simulink model "AE_sunroof_project"  (R2022b)
settings: Solver=VariableStepAuto  StartTime=0.0  StopTime=inf  RelTol=1e-3
libraries: simulink x3
settings Model: Creator=VENKATESH  LastModifiedBy=VENKATESH

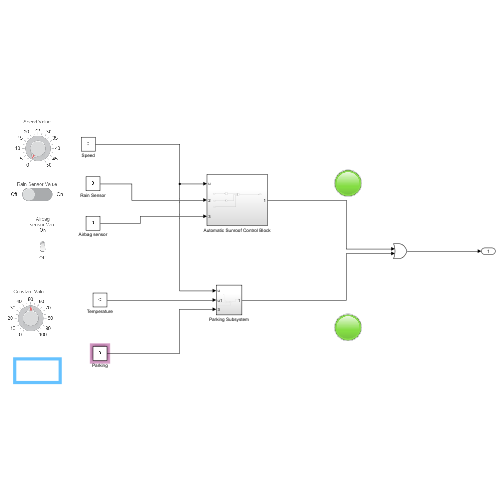
[thumbnail: Simulink's stored preview of the top-level diagram]
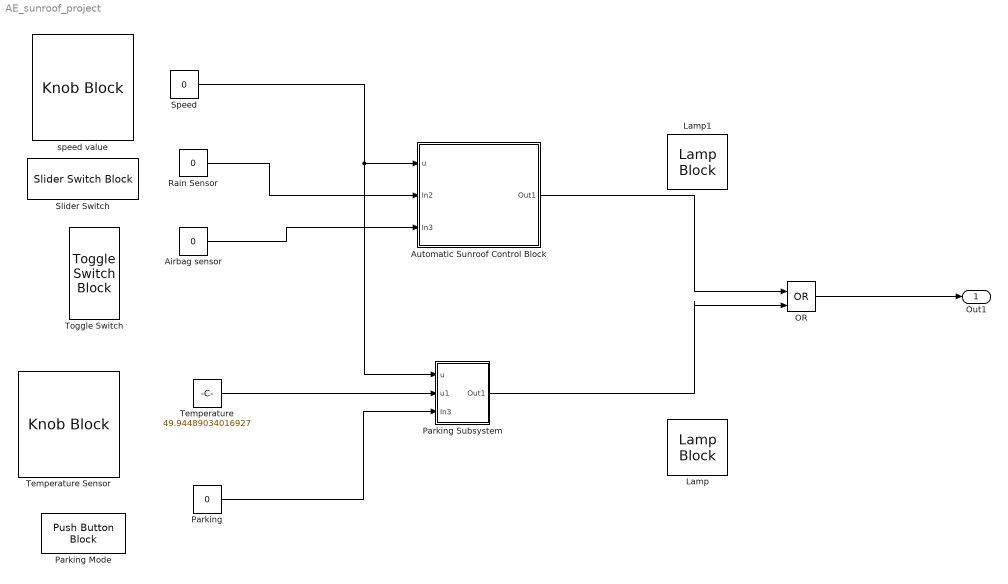
== system AE_sunroof_project ==
  Airbag sensor : Constant  Value=0
  Automatic Sunroof Control Block : Subsystem
  Lamp : LampBlock  LabelPosition=Hide
  Lamp1 : LampBlock  LabelPosition=Hide
  OR : Logic  Operator=OR  IconShape=distinctive  AllPortsSameDT=off  OutDataTypeStr=boolean
  Parking : Constant  Value=0
  Parking Mode : PushButtonBlock  ButtonType=Latch  OffValue=0.000000
  Parking Subsystem : Subsystem
  Rain Sensor : Constant  Value=0
  Slider Switch : SliderSwitchBlock
      settings: Values={{'Off', 'On'}, [0 1]}
  Speed : Constant  Value=0
  Temperature : Constant  Value=49.94489034016927
  Temperature Sensor : KnobBlock
  Toggle Switch : ToggleSwitchBlock
      settings: Values={{'Off', 'On'}, [0 1]}
  speed value : KnobBlock  ScaleMax=50
  Out1 : Outport
  wires:
  Speed/1 -> Parking Subsystem/1(u), Automatic Sunroof Control Block/1(u)
  Rain Sensor/1 -> Automatic Sunroof Control Block/2(In2)
  Airbag sensor/1 -> Automatic Sunroof Control Block/3(In3)
  Automatic Sunroof Control Block/1(Out1) -> OR/1
  OR/1 -> Out1/1
  Temperature/1 -> Parking Subsystem/2(u1)
  Parking/1 -> Parking Subsystem/3(In3)
  Parking Subsystem/1(Out1) -> OR/2

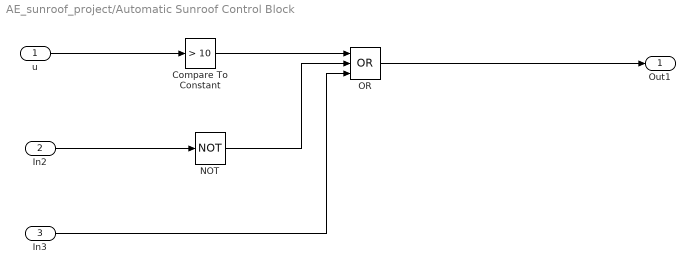
== system AE_sunroof_project/Automatic Sunroof Control Block ==
  u : Inport
  In2 : Inport  Port=2
  In3 : Inport  Port=3
  Compare To Constant : simulink/Logic and Bit Operations/Compare To Constant  relop=>  const=10  OutDataTypeStr=boolean
  NOT : Logic  Operator=NOT  IconShape=distinctive  AllPortsSameDT=off  OutDataTypeStr=boolean
  OR : Logic  Operator=OR  Inputs=3  IconShape=distinctive  AllPortsSameDT=off  OutDataTypeStr=boolean
  Out1 : Outport
  wires:
  In3/1 -> OR/3
  Compare To Constant/1 -> OR/1
  NOT/1 -> OR/2
  u/1 -> Compare To Constant/1
  In2/1 -> NOT/1
  OR/1 -> Out1/1

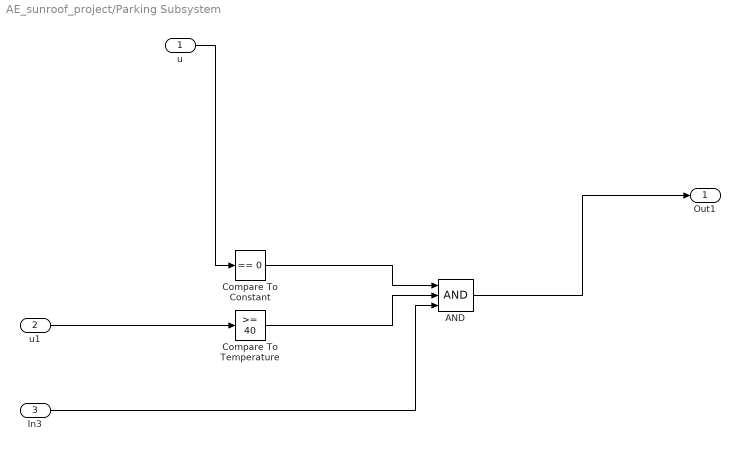
== system AE_sunroof_project/Parking Subsystem ==
  u : Inport
  u1 : Inport  Port=2
  In3 : Inport  Port=3
  AND : Logic  Inputs=3  IconShape=distinctive  AllPortsSameDT=off  OutDataTypeStr=boolean
  Compare To Constant : simulink/Logic and Bit Operations/Compare To Constant  relop===  const=0  OutDataTypeStr=boolean
  Compare To Temperature : simulink/Logic and Bit Operations/Compare To Constant  relop=>=  const=40  OutDataTypeStr=boolean
  Out1 : Outport
  wires:
  Compare To Constant/1 -> AND/1
  Compare To Temperature/1 -> AND/2
  u1/1 -> Compare To Temperature/1
  AND/1 -> Out1/1
  u/1 -> Compare To Constant/1
  In3/1 -> AND/3
